simulink model "main_sim_claw_main_sf"  (Simulink 7.2)
settings: Solver=ode2  SolverMode=SingleTasking  StartTime=0.0  StopTime=tsim_max  FixedStep=dtsim  RelTol=1e-3
StopFcn:
  | %mkplt
undefined symbols (not defined in the file): assertion_time, dtsim, MACH, MACH_gain_mat, MACH_mass_IC, MACH_pos_IC, MACH_pqr_Bmat_IC, MACH_pqr_u_IC, MACH_quat_IC, MACH_throttle_IC, MACH_U_nom_IC, MACH_vel_Bmat_IC, MACH_vel_cvdnom_IC, MACH_vel_IC, MACH_vel_uold_IC, max_LOS_rate, target_pos_IC, target_vel_IC, trac_params, u_llim, u_ulim, use_variable_mass, x_trac_IC
libraries: model_lib x8, mach_lib x5, simulink x3, models x1, utility_lib x1
(part 1 of 2)
CloseFcn:
  | rtwprivate ssgencode ModelCloseRequest main
settings Model: Creator=E183308  LastModifiedBy=E183308  ModifiedComment=E700252 -- Tue Nov 11 13:33:23 2003 -- Version 1.2477  TunableVars=MACH_U_nom_IC,MACH_gain_mat,MACH_mass_IC,MACH_pos_IC,MACH_pqr_Bmat_IC,MACH_pqr_u_IC,MACH_quat_IC,MACH_throttle_IC,MACH_vel_Bmat_IC,MACH_vel_IC,MACH_vel_cvdnom_IC,MACH_vel_uold_IC  TunableVarsStorageClass=Auto,Auto,Auto,Auto,Auto,Auto,Auto,Auto,Auto,Auto,Auto,Auto  TunableVarsTypeQualifier=,,,,,,,,,,,  BufferReuse=off
settings DataIOCC: LimitDataPoints=off  SaveOutput=off  SaveTime=off  SignalLoggingName=sigsOut
settings OptimizationCC: BlockReduction=off  BooleanDataType=off  BufferReuse=off  EnforceIntegerDowncast=off  FoldNonRolledExpr=off  InitFltsAndDblsToZero=on
settings DebuggingCC: SaveWithParameterizedLinksMsg=none  SignalResolutionControl=TryResolveAllWithWarning  SolverPrmCheckMsg=none  InheritedTsInSrcMsg=none  MultiTaskDSMMsg=warning  MultiTaskCondExecSysMsg=none  StrictBusMsg=ErrorLevel1
settings HardwareCC: TargetEndianess=LittleEndian  TargetHWDeviceType=MATLAB Host  ProdEqTarget=off
settings SFSimCC: SFSimEcho=off
settings RTWCC: SystemTargetFile=rtwsfcn.tlc  TemplateMakefile=rtwsfcn_default_tmf  Description=S-function Target  ProcessScript=rtwsfcn_make_rtw_hook  IncludeERTFirstTime=on
settings STFCustomTargetCC: TargetFcnLib=ansi_tfl_tmw.mat  ModelReferenceCompliant=off  SystemTargetFile=rtwsfcn.tlc
settings CustomProperty: Value=on

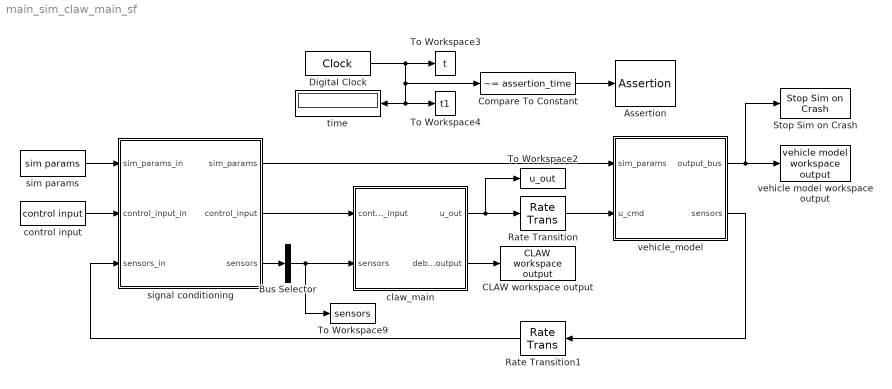
== system main_sim_claw_main_sf ==
  Assertion : Assertion  Enabled=on  AssertionFailFcn=assertioncb  StopWhenAssertionFail=off
  Bus Selector : BusSelector  OutputSignals=pqr,NED_dot,latlonh,e,accels_cg,nav_ok,u_meas,NED_wind,seeker  OutputAsBus=on
  CLAW workspace output : mach_lib/CLAW workspace output  SystemSampleTime=-1
  Compare To Constant : simulink/Logic and Bit Operations/Compare To Constant  SystemSampleTime=-1  relop=~=  const=assertion_time  LogicOutDataTypeMode=boolean  ZeroCross=off
  Digital Clock : DigitalClock  SampleTime=dtsim
  Rate Transition : RateTransition  X0=MACH_U_nom_IC
  Rate Transition1 : RateTransition  Orientation=left  OutPortSampleTime=MACH.dt
  Stop Sim on Crash : mach_lib/Stop Sim on Crash  SystemSampleTime=-1
  To Workspace2 : ToWorkspace  VariableName=u_out  SampleTime=MACH.dt  SaveFormat=Array
  To Workspace3 : ToWorkspace  VariableName=t  SampleTime=dtsim  SaveFormat=Array
  To Workspace4 : ToWorkspace  VariableName=t1  SampleTime=MACH.dt  SaveFormat=Array
  To Workspace9 : ToWorkspace  VariableName=sensors  SampleTime=MACH.dt  SaveFormat=Array
      settings: MaxDataPoints=1
  claw_main : Subsystem  mask{prm_to_disp=[1..10], sfcnParam1=MACH_U_nom_IC, sfcnParam2=MACH_gain_mat, sfcnParam3=MACH_mass_IC, sfcnParam4=MACH_pos_IC, sfcnParam5=MACH_pqr_Bmat_IC, sfcnParam6=MACH_pqr_u_IC, sfcnParam7=MACH_quat_IC, sfcnParam8=MACH_throttle_IC, sfcnParam9=MACH_vel_Bmat_IC, sfcnParam10=MACH_vel_IC, sfcnParam11=MACH_vel_cvdnom_IC, sfcnParam12=MACH_vel_uold_IC}
      mask prompts: prm_to_disp "Display S-function Parameters:"; sfcnParam1 "MACH_U_nom_IC:"; sfcnParam2 "MACH_gain_mat:"; sfcnParam3 "MACH_mass_IC:"; sfcnParam4 "MACH_pos_IC:"; sfcnParam5 "MACH_pqr_Bmat_IC:"; sfcnParam6 "MACH_pqr_u_IC:"; sfcnParam7 "MACH_quat_IC:"; sfcnParam8 "MACH_throttle_IC:"; sfcnParam9 "MACH_vel_Bmat_IC:"; sfcnParam10 "MACH_vel_IC:"; sfcnParam11 "MACH_vel_cvdnom_IC:"; sfcnParam12 "MACH_vel_uold_IC:"
      mask help: Real-Time Workshop generated S-function.
      mask Help: eval('feval(''rtwprivate'',''rtwhelpview'',''rtw_sfcn_block'')');
      mask StyleString: popup([1..10]|[11..12]),edit,edit,edit,edit,edit,edit,edit,edit,edit,edit,edit,edit
      mask CallbackString: slmaskprmdispcntrl(gcbh)||||||||||||
  control input : mach_lib/control input  SystemSampleTime=MACH.dt
  signal conditioning : Subsystem
  sim params : mach_lib/sim params  SystemSampleTime=-1
  time : Display
  vehicle model workspace output : mach_lib/vehicle model workspace output  SystemSampleTime=-1
  vehicle_model : Subsystem  TreatAsAtomicUnit=on
  wires:
  Digital Clock/1 -> To Workspace3/1, time/1, To Workspace4/1, Compare To Constant/1
  claw_main/1(u_out) -> Rate Transition/1, To Workspace2/1
  vehicle_model/2(sensors) -> Rate Transition1/1
  claw_main/2(debug_output) -> CLAW workspace output/1
  Rate Transition/1 -> vehicle_model/2(u_cmd)
  Bus Selector/1 -> To Workspace9/1, claw_main/2(sensors)
  vehicle_model/1(output_bus) -> vehicle model workspace output/1, Stop Sim on Crash/1
  Rate Transition1/1 -> signal conditioning/3(sensors_in)
  signal conditioning/3(sensors) -> Bus Selector/1
  signal conditioning/2(control_input) -> claw_main/1(control_input)
  control input/1 -> signal conditioning/2(control_input_in)
  sim params/1 -> signal conditioning/1(sim_params_in)
  signal conditioning/1(sim_params) -> vehicle_model/1(sim_params)
  Compare To Constant/1 -> Assertion/1

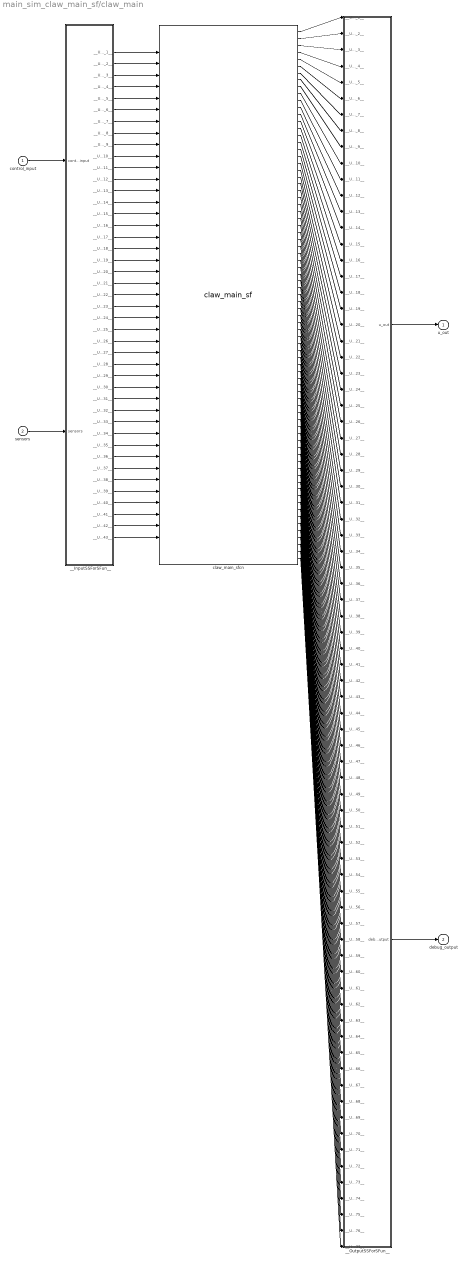
== system main_sim_claw_main_sf/claw_main ==
  control_input : Inport  OutDataType=sfix(16)  OutScaling=2^0
      settings: BusObject=control_input_bus
  sensors : Inport  Port=2  OutDataType=sfix(16)  OutScaling=2^0
  __InputSSForSFun__ : Subsystem
  __OutputSSForSFun__ : Subsystem
  claw_main_sfcn : S-Function  FunctionName=claw_main_sf  Parameters=sfcnParam1, sfcnParam2, sfcnParam3, sfcnParam4, sfcnParam5, sfcnParam6, sfcnParam7, sfcnParam8, sfcnParam9, sfcnParam10, sfcnParam11, sfcnParam12  SFunctionModules=""  EnableBusSupport=off  mask{rtw_sf_name=claw_main_sf, showVar=off, prm_to_disp=[1..10], sfcnParam1=sfcnParam1, sfcnParam2=sfcnParam2, sfcnParam3=sfcnParam3, sfcnParam4=sfcnParam4, sfcnParam5=sfcnParam5, sfcnParam6=sfcnParam6, sfcnParam7=sfcnParam7, sfcnParam8=sfcnParam8, sfcnParam9=sfcnParam9, sfcnParam10=sfcnParam10, sfcnParam11=sfcnParam11, sfcnParam12=sfcnParam12}
      mask prompts: rtw_sf_name "Generated S-function name (model_sf):"; showVar "Show module list"; prm_to_disp "Display S-function Parameters:"; sfcnParam1 "MACH_U_nom_IC:"; sfcnParam2 "MACH_gain_mat:"; sfcnParam3 "MACH_mass_IC:"; sfcnParam4 "MACH_pos_IC:"; sfcnParam5 "MACH_pqr_Bmat_IC:"; sfcnParam6 "MACH_pqr_u_IC:"; sfcnParam7 "MACH_quat_IC:"; sfcnParam8 "MACH_throttle_IC:"; sfcnParam9 "MACH_vel_Bmat_IC:"; sfcnParam10 "MACH_vel_IC:"; sfcnParam11 "MACH_vel_cvdnom_IC:"; sfcnParam12 "MACH_vel_uold_IC:"
      mask help: Real-Time Workshop generated S-function.
      mask init:
      | displist = '';
      | if ~strcmp(get_param(gcb, 'FunctionName'), rtw_sf_name);
      |   set_param(gcb, 'FunctionName', rtw_sf_name);
      | end
      | % Check if we are generating RTW code
      | rtw_mode = false;
      | if strcmpi(get_param(bdroot(gcb),'SimulationStatus'),'Initializing')
      | 	rtw_mode = strcmpi(get_param(bdroot(gcb),'BuildingRTWCode'),'on') && ...
      | 		~strcmpi(get_param(bdroot(gcb),'TargetStyle'),'SimulationTarget');
      | end
      | if showVar || rtw_mode
      | 	if exist('rtwsfunc') == 2 | exist('rtwsfunc') == 6
      | 		tmplist = rtwsfunc(rtw_sf_name,gcb);
      | 		tmplist = ['\nList of Modules:\n', tmplist];
      | 	elseif showVar
      | 		tmplist = '\nList of Modules:\nRTW not licensed\n';
      |  	end
      | end
      | if showVar
      |   displist = tmplist;
      | end
      settings: CopyFcn=|
      | if ~strcmp(get_param(gcb,'Linkstatus'),'none') && ...
      | ~strcmp(get_param(gcb,'Linkstatus'),'implicit')
      |   set_param(gcb,'LinkStatus','none');
      | end
      mask Help: eval('feval(''rtwprivate'',''rtwhelpview'',''rtw_sfcn_block'')');
      mask StyleString: edit,checkbox,popup([1..10]|[11..12]),edit,edit,edit,edit,edit,edit,edit,edit,edit,edit,edit,edit
      mask CallbackString: ||slmaskprmdispcntrl(gcbh)||||||||||||
      mask Display:
      | port_label('input',1,'command');
      | port_label('input',2,'full_surf_cmd');
      | port_label('input',3,'full_surf_ulim');
      | port_label('input',4,'full_surf_llim');
      | port_label('input',5,'full_surf_urlim');
      | port_label('input',6,'full_surf_lrlim');
      | port_label('input',7,'full_surf_lock');
      | port_label('input',8,'full_surf_pref_select');
      | port_label('input',9,'full_surf_pref');
      | port_label('input',10,'full_surf_pref_wght');
      | port_label('input',11,'CLAW_mode');
      | port_label('input',12,'engaged_sw');
      | port_label('input',13,'accel_submode');
      | port_label('input',14,'pre_takeoff_sw');
      | port_label('input',15,'reset_pos_sw');
      | port_label('input',16,'wind_est_sw');
      | port_label('input',17,'llh_input_sw');
      | port_label('input',18,'int_reset_sw');
      | port_label('input',19,'att_type');
      | port_label('input',20,'cam_rate_cmd_sw');
      | port_label('input',21,'full_surf_cmd_sw');
      | port_label('input',22,'enable_homing_sw');
      | port_label('input',23,'att_rate_cmd_sw');
      | port_label('input',24,'nav_enable_sw');
      | port_label('input',25,'enable_bb_sw');
      | port_label('input',26,'gain_set_sw');
      | port_label('input',27,'use_held_aero_obac_sw');
      | port_label('input',28,'Isp_sl');
      | port_label('input',29,'Isp_vacuum');
      | port_label('input',30,'throt_to_ff');
      | port_label('input',31,'pqr');
      | port_label('input',32,'NED_dot');
      | port_label('input',33,'latlonh');
      | port_label('input',34,'e');
      | port_label('input',35,'accels_cg');
      | port_label('input',36,'nav_ok');
      | port_label('input',37,'u_meas');
      | port_label('input',38,'NED_wind');
      | port_label('input',39,'LOS_rate');
      | port_label('input',40,'azimuth');
      | port_label('input',41,'elevation');
      | port_label('input',42,'Rground');
      | port_label('input',43,'Rslant');
      | port_label('output',1,'u_out');
      | port_label('output',2,'commandb');
      | port_label('output',3,'full_surf_cmdb');
      | port_label('output',4,'full_surf_ulimb');
      | port_label('output',5,'full_surf_llimb');
      | port_label('output',6,'full_surf_urlimb');
      | port_label('output',7,'full_surf_lrlimb');
      | port_label('output',8,'full_surf_lockb');
      | port_label('output',9,'full_surf_pref_selectb');
      | port_label('output',10,'full_surf_prefb');
      | port_label('output',11,'full_surf_pref_wghtb');
      | port_label('output',12,'CLAW_modeb');
      | port_label('output',13,'engaged_swb');
      | port_label('output',14,'accel_submodeb');
      | port_label('output',15,'pre_takeoff_swb');
      | port_label('output',16,'reset_pos_swb');
      | port_label('output',17,'wind_est_swb');
      | port_label('output',18,'llh_input_swb');
      | port_label('output',19,'int_reset_swb');
      | port_label('output',20,'att_typeb');
      | port_label('output',21,'cam_rate_cmd_swb');
      | port_label('output',22,'full_surf_cmd_swb');
      | port_label('output',23,'enable_homing_swb');
      | port_label('output',24,'att_rate_cmd_swb');
      | port_label('output',25,'nav_enable_swb');
      | port_label('output',26,'enable_bb_swb');
      | port_label('output',27,'gain_set_swb');
      | port_label('output',28,'use_held_aero_obac_swb');
      | port_label('output',29,'Isp_slb');
      | port_label('output',30,'Isp_vacuumb');
      | port_label('output',31,'throt_to_ffb');
      | port_label('output',32,'cvdex_smn');
      | port_label('output',33,'lambda');
      | port_label('output',34,'solve_dat');
      | port_label('output',35,'cvdex');
      | port_label('output',36,'cvc');
      | port_label('output',37,'integ');
      | port_label('output',38,'cv');
      | port_label('output',39,'cvdnom');
      | port_label('output',40,'Bmat');
      | port_label('output',41,'u_ulim');
      | port_label('output',42,'u_llim');
      | port_label('output',43,'u_pref');
      | port_label('output',44,'bb_debug');
      | port_label('output',45,'cvdexb');
      | port_label('output',46,'integb');
      | port_label('output',47,'cvcb');
      | port_label('output',48,'cvb');
      | port_label('output',49,'tiltcam_cmds');
      | port_label('output',50,'rpy_cmds');
      | port_label('output',51,'mab_cmds');
      | port_label('output',52,'cvdexa');
      | port_label('output',53,'lambdab');
      | port_label('output',54,'solve_datb');
      | port_label('output',55,'intega');
      | port_label('output',56,'cvca');
      | port_label('output',57,'cva');
      | port_label('output',58,'cvdnomb');
      | port_label('output',59,'Bmatb');
      | port_label('output',60,'Bmat_fltpath');
      | port_label('output',61,'u_ulimb');
      | port_label('output',62,'u_llimb');
      | port_label('output',63,'cvdex_fltpath');
      | port_label('output',64,'cvdexc');
      | port_label('output',65,'integc');
      | port_label('output',66,'cvcc');
      | port_label('output',67,'cvd');
      | port_label('output',68,'cvdex_fltpathb');
      | port_label('output',69,'w_est');
      | port_label('output',70,'NED_wind_ex');
      | port_label('output',71,'uvw_wind');
      | port_label('output',72,'uvw_rw_est');
      | port_label('output',73,'accels');
      | port_label('output',74,'att_typea');
      | port_label('output',75,'mass');
      | port_label('output',76,'enable_bb');
      | port_label('output',77,'gain_set');
  u_out : Outport  OutDataType=sfix(16)  OutScaling=2^0
  debug_output : Outport  Port=2  OutDataType=sfix(16)  OutScaling=2^0
  wires:
  control_input/1 -> __InputSSForSFun__/1(control_input)
  sensors/1 -> __InputSSForSFun__/2(sensors)
  __InputSSForSFun__/1(__UniqueOutportName__1__) -> claw_main_sfcn/1
  __InputSSForSFun__/2(__UniqueOutportName__2__) -> claw_main_sfcn/2
  __InputSSForSFun__/3(__UniqueOutportName__3__) -> claw_main_sfcn/3
  __InputSSForSFun__/4(__UniqueOutportName__4__) -> claw_main_sfcn/4
  __InputSSForSFun__/5(__UniqueOutportName__5__) -> claw_main_sfcn/5
  __InputSSForSFun__/6(__UniqueOutportName__6__) -> claw_main_sfcn/6
  __InputSSForSFun__/7(__UniqueOutportName__7__) -> claw_main_sfcn/7
  __InputSSForSFun__/8(__UniqueOutportName__8__) -> claw_main_sfcn/8
  __InputSSForSFun__/9(__UniqueOutportName__9__) -> claw_main_sfcn/9
  __InputSSForSFun__/10(__UniqueOutportName__10__) -> claw_main_sfcn/10
  __InputSSForSFun__/11(__UniqueOutportName__11__) -> claw_main_sfcn/11
  __InputSSForSFun__/12(__UniqueOutportName__12__) -> claw_main_sfcn/12
  __InputSSForSFun__/13(__UniqueOutportName__13__) -> claw_main_sfcn/13
  __InputSSForSFun__/14(__UniqueOutportName__14__) -> claw_main_sfcn/14
  __InputSSForSFun__/15(__UniqueOutportName__15__) -> claw_main_sfcn/15
  __InputSSForSFun__/16(__UniqueOutportName__16__) -> claw_main_sfcn/16
  __InputSSForSFun__/17(__UniqueOutportName__17__) -> claw_main_sfcn/17
  __InputSSForSFun__/18(__UniqueOutportName__18__) -> claw_main_sfcn/18
  __InputSSForSFun__/19(__UniqueOutportName__19__) -> claw_main_sfcn/19
  __InputSSForSFun__/20(__UniqueOutportName__20__) -> claw_main_sfcn/20
  __InputSSForSFun__/21(__UniqueOutportName__21__) -> claw_main_sfcn/21
  __InputSSForSFun__/22(__UniqueOutportName__22__) -> claw_main_sfcn/22
  __InputSSForSFun__/23(__UniqueOutportName__23__) -> claw_main_sfcn/23
  __InputSSForSFun__/24(__UniqueOutportName__24__) -> claw_main_sfcn/24
  __InputSSForSFun__/25(__UniqueOutportName__25__) -> claw_main_sfcn/25
  __InputSSForSFun__/26(__UniqueOutportName__26__) -> claw_main_sfcn/26
  __InputSSForSFun__/27(__UniqueOutportName__27__) -> claw_main_sfcn/27
  __InputSSForSFun__/28(__UniqueOutportName__28__) -> claw_main_sfcn/28
  __InputSSForSFun__/29(__UniqueOutportName__29__) -> claw_main_sfcn/29
  __InputSSForSFun__/30(__UniqueOutportName__30__) -> claw_main_sfcn/30
  __InputSSForSFun__/31(__UniqueOutportName__31__) -> claw_main_sfcn/31
  __InputSSForSFun__/32(__UniqueOutportName__32__) -> claw_main_sfcn/32
  __InputSSForSFun__/33(__UniqueOutportName__33__) -> claw_main_sfcn/33
  __InputSSForSFun__/34(__UniqueOutportName__34__) -> claw_main_sfcn/34
  __InputSSForSFun__/35(__UniqueOutportName__35__) -> claw_main_sfcn/35
  __InputSSForSFun__/36(__UniqueOutportName__36__) -> claw_main_sfcn/36
  __InputSSForSFun__/37(__UniqueOutportName__37__) -> claw_main_sfcn/37
  __InputSSForSFun__/38(__UniqueOutportName__38__) -> claw_main_sfcn/38
  __InputSSForSFun__/39(__UniqueOutportName__39__) -> claw_main_sfcn/39
  __InputSSForSFun__/40(__UniqueOutportName__40__) -> claw_main_sfcn/40
  __InputSSForSFun__/41(__UniqueOutportName__41__) -> claw_main_sfcn/41
  __InputSSForSFun__/42(__UniqueOutportName__42__) -> claw_main_sfcn/42
  __InputSSForSFun__/43(__UniqueOutportName__43__) -> claw_main_sfcn/43
  claw_main_sfcn/1 -> __OutputSSForSFun__/1(__UniqueInportName__1__)
  claw_main_sfcn/2 -> __OutputSSForSFun__/2(__UniqueInportName__2__)
  claw_main_sfcn/3 -> __OutputSSForSFun__/3(__UniqueInportName__3__)
  claw_main_sfcn/4 -> __OutputSSForSFun__/4(__UniqueInportName__4__)
  claw_main_sfcn/5 -> __OutputSSForSFun__/5(__UniqueInportName__5__)
  claw_main_sfcn/6 -> __OutputSSForSFun__/6(__UniqueInportName__6__)
  claw_main_sfcn/7 -> __OutputSSForSFun__/7(__UniqueInportName__7__)
  claw_main_sfcn/8 -> __OutputSSForSFun__/8(__UniqueInportName__8__)
  claw_main_sfcn/9 -> __OutputSSForSFun__/9(__UniqueInportName__9__)
  claw_main_sfcn/10 -> __OutputSSForSFun__/10(__UniqueInportName__10__)
  claw_main_sfcn/11 -> __OutputSSForSFun__/11(__UniqueInportName__11__)
  claw_main_sfcn/12 -> __OutputSSForSFun__/12(__UniqueInportName__12__)
  claw_main_sfcn/13 -> __OutputSSForSFun__/13(__UniqueInportName__13__)
  claw_main_sfcn/14 -> __OutputSSForSFun__/14(__UniqueInportName__14__)
  claw_main_sfcn/15 -> __OutputSSForSFun__/15(__UniqueInportName__15__)
  claw_main_sfcn/16 -> __OutputSSForSFun__/16(__UniqueInportName__16__)
  claw_main_sfcn/17 -> __OutputSSForSFun__/17(__UniqueInportName__17__)
  claw_main_sfcn/18 -> __OutputSSForSFun__/18(__UniqueInportName__18__)
  claw_main_sfcn/19 -> __OutputSSForSFun__/19(__UniqueInportName__19__)
  claw_main_sfcn/20 -> __OutputSSForSFun__/20(__UniqueInportName__20__)
  claw_main_sfcn/21 -> __OutputSSForSFun__/21(__UniqueInportName__21__)
  claw_main_sfcn/22 -> __OutputSSForSFun__/22(__UniqueInportName__22__)
  claw_main_sfcn/23 -> __OutputSSForSFun__/23(__UniqueInportName__23__)
  claw_main_sfcn/24 -> __OutputSSForSFun__/24(__UniqueInportName__24__)
  claw_main_sfcn/25 -> __OutputSSForSFun__/25(__UniqueInportName__25__)
  claw_main_sfcn/26 -> __OutputSSForSFun__/26(__UniqueInportName__26__)
  claw_main_sfcn/27 -> __OutputSSForSFun__/27(__UniqueInportName__27__)
  claw_main_sfcn/28 -> __OutputSSForSFun__/28(__UniqueInportName__28__)
  claw_main_sfcn/29 -> __OutputSSForSFun__/29(__UniqueInportName__29__)
  claw_main_sfcn/30 -> __OutputSSForSFun__/30(__UniqueInportName__30__)
  claw_main_sfcn/31 -> __OutputSSForSFun__/31(__UniqueInportName__31__)
  claw_main_sfcn/32 -> __OutputSSForSFun__/32(__UniqueInportName__32__)
  claw_main_sfcn/33 -> __OutputSSForSFun__/33(__UniqueInportName__33__)
  claw_main_sfcn/34 -> __OutputSSForSFun__/34(__UniqueInportName__34__)
  claw_main_sfcn/35 -> __OutputSSForSFun__/35(__UniqueInportName__35__)
  claw_main_sfcn/36 -> __OutputSSForSFun__/36(__UniqueInportName__36__)
  claw_main_sfcn/37 -> __OutputSSForSFun__/37(__UniqueInportName__37__)
  claw_main_sfcn/38 -> __OutputSSForSFun__/38(__UniqueInportName__38__)
  claw_main_sfcn/39 -> __OutputSSForSFun__/39(__UniqueInportName__39__)
  claw_main_sfcn/40 -> __OutputSSForSFun__/40(__UniqueInportName__40__)
  claw_main_sfcn/41 -> __OutputSSForSFun__/41(__UniqueInportName__41__)
  claw_main_sfcn/42 -> __OutputSSForSFun__/42(__UniqueInportName__42__)
  claw_main_sfcn/43 -> __OutputSSForSFun__/43(__UniqueInportName__43__)
  claw_main_sfcn/44 -> __OutputSSForSFun__/44(__UniqueInportName__44__)
  claw_main_sfcn/45 -> __OutputSSForSFun__/45(__UniqueInportName__45__)
  claw_main_sfcn/46 -> __OutputSSForSFun__/46(__UniqueInportName__46__)
  claw_main_sfcn/47 -> __OutputSSForSFun__/47(__UniqueInportName__47__)
  claw_main_sfcn/48 -> __OutputSSForSFun__/48(__UniqueInportName__48__)
  claw_main_sfcn/49 -> __OutputSSForSFun__/49(__UniqueInportName__49__)
  claw_main_sfcn/50 -> __OutputSSForSFun__/50(__UniqueInportName__50__)
  claw_main_sfcn/51 -> __OutputSSForSFun__/51(__UniqueInportName__51__)
  claw_main_sfcn/52 -> __OutputSSForSFun__/52(__UniqueInportName__52__)
  claw_main_sfcn/53 -> __OutputSSForSFun__/53(__UniqueInportName__53__)
  claw_main_sfcn/54 -> __OutputSSForSFun__/54(__UniqueInportName__54__)
  claw_main_sfcn/55 -> __OutputSSForSFun__/55(__UniqueInportName__55__)
  claw_main_sfcn/56 -> __OutputSSForSFun__/56(__UniqueInportName__56__)
  claw_main_sfcn/57 -> __OutputSSForSFun__/57(__UniqueInportName__57__)
  claw_main_sfcn/58 -> __OutputSSForSFun__/58(__UniqueInportName__58__)
  claw_main_sfcn/59 -> __OutputSSForSFun__/59(__UniqueInportName__59__)
  claw_main_sfcn/60 -> __OutputSSForSFun__/60(__UniqueInportName__60__)
  claw_main_sfcn/61 -> __OutputSSForSFun__/61(__UniqueInportName__61__)
  claw_main_sfcn/62 -> __OutputSSForSFun__/62(__UniqueInportName__62__)
  claw_main_sfcn/63 -> __OutputSSForSFun__/63(__UniqueInportName__63__)
  claw_main_sfcn/64 -> __OutputSSForSFun__/64(__UniqueInportName__64__)
  claw_main_sfcn/65 -> __OutputSSForSFun__/65(__UniqueInportName__65__)
  claw_main_sfcn/66 -> __OutputSSForSFun__/66(__UniqueInportName__66__)
  claw_main_sfcn/67 -> __OutputSSForSFun__/67(__UniqueInportName__67__)
  claw_main_sfcn/68 -> __OutputSSForSFun__/68(__UniqueInportName__68__)
  claw_main_sfcn/69 -> __OutputSSForSFun__/69(__UniqueInportName__69__)
  claw_main_sfcn/70 -> __OutputSSForSFun__/70(__UniqueInportName__70__)
  claw_main_sfcn/71 -> __OutputSSForSFun__/71(__UniqueInportName__71__)
  claw_main_sfcn/72 -> __OutputSSForSFun__/72(__UniqueInportName__72__)
  claw_main_sfcn/73 -> __OutputSSForSFun__/73(__UniqueInportName__73__)
  claw_main_sfcn/74 -> __OutputSSForSFun__/74(__UniqueInportName__74__)
  claw_main_sfcn/75 -> __OutputSSForSFun__/75(__UniqueInportName__75__)
  claw_main_sfcn/76 -> __OutputSSForSFun__/76(__UniqueInportName__76__)
  claw_main_sfcn/77 -> __OutputSSForSFun__/77(__UniqueInportName__77__)
  __OutputSSForSFun__/1(u_out) -> u_out/1
  __OutputSSForSFun__/2(debug_output) -> debug_output/1

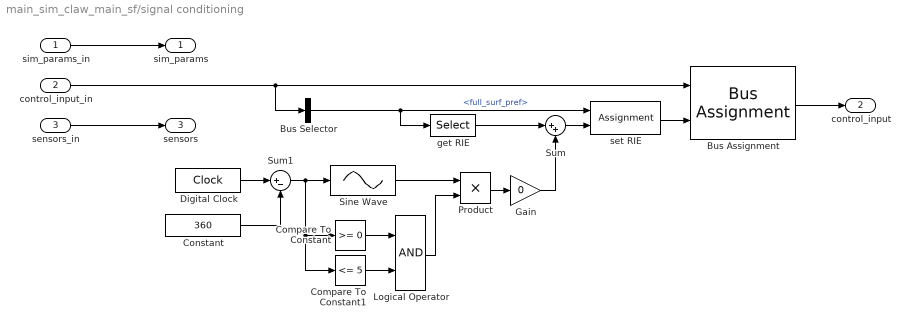
== system main_sim_claw_main_sf/signal conditioning ==
  sim_params_in : Inport  OutDataType=sfix(16)  OutScaling=2^0
  control_input_in : Inport  Port=2  OutDataType=sfix(16)  OutScaling=2^0
  sensors_in : Inport  Port=3  OutDataType=sfix(16)  OutScaling=2^0
  Bus Assignment : BusAssignment  AssignedSignals=full_surf.full_surf_pref
  Bus Selector : BusSelector  OutputSignals=full_surf.full_surf_pref
  Compare To Constant : simulink/Logic and Bit Operations/Compare To Constant  SystemSampleTime=-1  relop=>=  const=0  LogicOutDataTypeMode=boolean  ZeroCross=off
  Compare To Constant1 : simulink/Logic and Bit Operations/Compare To Constant  SystemSampleTime=-1  relop=<=  const=5  LogicOutDataTypeMode=boolean  ZeroCross=off
  Constant : Constant  Value=360  OutDataType=sfix(16)  OutScaling=2^0
  Digital Clock : DigitalClock  SampleTime=MACH.dt
  Gain : Gain  Gain=0  ParameterDataType=sfix(16)  ParameterScaling=2^0  OutDataType=sfix(16)  OutScaling=2^0
  Logical Operator : Logic  AllPortsSameDT=off
  Product : Product  OutDataType=sfix(16)  OutScaling=2^0  RndMeth=Zero
  Sine Wave : Sin  TimeSource=Use external signal  Amplitude=5  Frequency=2*pi  SampleTime=0
  Sum : Sum  Inputs=|++  OutDataType=sfix(16)  OutScaling=2^0
  Sum1 : Sum  Inputs=|+-  OutDataType=sfix(16)  OutScaling=2^0
  get RIE : Selector  InputPortWidth=MACH.num_u  IndexOptions=Index vector (dialog)  Indices=MACH.vane_idx(1)  OutputSizes=1
  set RIE : Assignment  IndexOptions=Index vector (dialog)  Indices=MACH.vane_idx(1)  OutputSizes=[1 1]
  sim_params : Outport  OutDataType=sfix(16)  OutScaling=2^0
  control_input : Outport  Port=2  OutDataType=sfix(16)  OutScaling=2^0
  sensors : Outport  Port=3  OutDataType=sfix(16)  OutScaling=2^0
  wires:
  sim_params_in/1 -> sim_params/1
  control_input_in/1 -> Bus Assignment/1, Bus Selector/1
  sensors_in/1 -> sensors/1
  set RIE/1 -> Bus Assignment/2
  Sum/1 -> set RIE/2
  Bus Selector/1 -> set RIE/1, get RIE/1  "<full_surf_pref>"
  get RIE/1 -> Sum/1
  Digital Clock/1 -> Sum1/1
  Constant/1 -> Sum1/2
  Sum1/1 -> Sine Wave/1, Compare To Constant/1, Compare To Constant1/1
  Compare To Constant/1 -> Logical Operator/1
  Compare To Constant1/1 -> Logical Operator/2
  Logical Operator/1 -> Product/2
  Sine Wave/1 -> Product/1
  Product/1 -> Gain/1
  Bus Assignment/1 -> control_input/1
  Gain/1 -> Sum/2

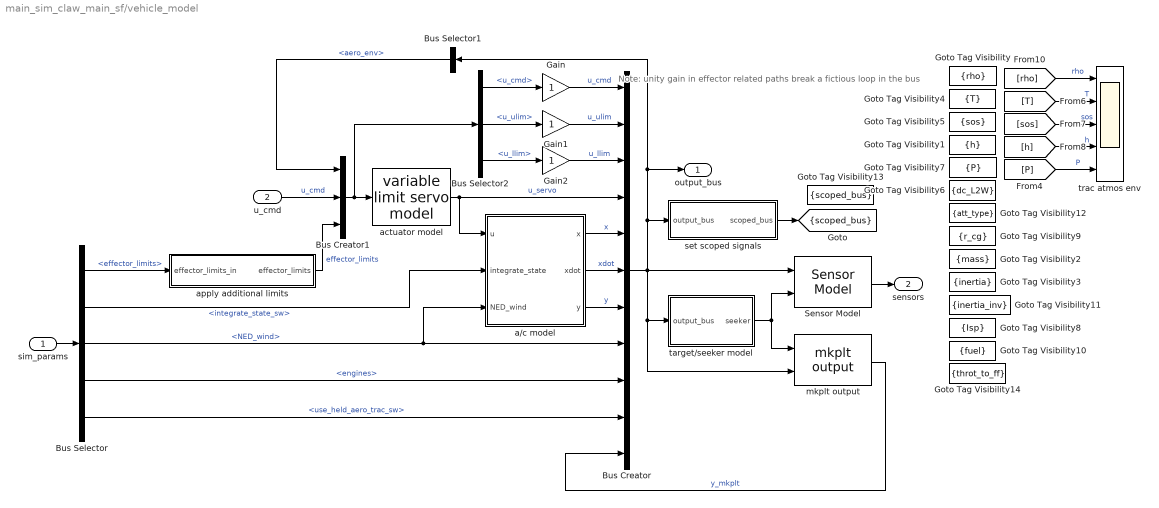
== system main_sim_claw_main_sf/vehicle_model ==
  note: Note: unity gain in effector related paths
      | break a fictious loop in the bus
  sim_params : Inport  OutDataType=sfix(16)  OutScaling=2^0
  u_cmd : Inport  Port=2  OutDataType=sfix(16)  OutScaling=2^0
  Bus Creator : BusCreator  Inputs=11
  Bus Creator1 : BusCreator  Inputs=3
  Bus Selector : BusSelector  OutputSignals=effector_limits,integrate_state_sw,NED_wind,engines,use_held_aero_trac_sw
  Bus Selector1 : BusSelector  Orientation=left  OutputSignals=y.aero_env
  Bus Selector2 : BusSelector  OutputSignals=u_cmd,effector_limits.u_ulim,effector_limits.u_llim
  Gain : Gain  ParameterDataType=sfix(16)  ParameterScaling=2^0  OutDataType=sfix(16)  OutScaling=2^0
  Gain1 : Gain  ParameterDataType=sfix(16)  ParameterScaling=2^0  OutDataType=sfix(16)  OutScaling=2^0
  Gain2 : Gain  ParameterDataType=sfix(16)  ParameterScaling=2^0  OutDataType=sfix(16)  OutScaling=2^0
  Goto Tag Visibility : GotoTagVisibility  GotoTag=rho
  Goto Tag Visibility1 : GotoTagVisibility  GotoTag=h
  Goto Tag Visibility10 : GotoTagVisibility  GotoTag=fuel
  Goto Tag Visibility11 : GotoTagVisibility  GotoTag=inertia_inv
  Goto Tag Visibility12 : GotoTagVisibility  GotoTag=att_type
  Goto Tag Visibility13 : GotoTagVisibility  GotoTag=scoped_bus
  Goto Tag Visibility14 : GotoTagVisibility  GotoTag=throt_to_ff
  Goto Tag Visibility2 : GotoTagVisibility  GotoTag=mass
  Goto Tag Visibility3 : GotoTagVisibility  GotoTag=inertia
  Goto Tag Visibility4 : GotoTagVisibility  GotoTag=T
  Goto Tag Visibility5 : GotoTagVisibility  GotoTag=sos
  Goto Tag Visibility6 : GotoTagVisibility  GotoTag=dc_L2W
  Goto Tag Visibility7 : GotoTagVisibility  GotoTag=P
  Goto Tag Visibility8 : GotoTagVisibility  GotoTag=Isp
  Goto Tag Visibility9 : GotoTagVisibility  GotoTag=r_cg
  Sensor Model : model_lib/Sensor Model  SystemSampleTime=-1
  a/c model : Subsystem
  actuator model : model_lib/variable limit servo model  SystemSampleTime=-1
  apply additional limits : Subsystem
  mkplt output : model_lib/mkplt output  SystemSampleTime=-1
  set scoped signals : Subsystem
  target/seeker model : Subsystem
  trac atmos env : Scope  NumInputPorts=5
      settings: YMin=-5~-5~-5~-5~-5  YMax=5~5~5~5~5
  output_bus : Outport  OutDataType=sfix(16)  OutScaling=2^0
  sensors : Outport  Port=2  OutDataType=sfix(16)  OutScaling=2^0
  tag scope: scoped_bus=scoped
  wires:
  actuator model/1 -> a/c model/1(u), Bus Creator/4  "u_servo"
  Sensor Model/1 -> sensors/1
  Bus Selector/3 -> Bus Creator/8, a/c model/3(NED_wind)  "<NED_wind>"
  [h] -> trac atmos env/4  "h"
  [sos] -> trac atmos env/3  "sos"
  [T] -> trac atmos env/2  "T"
  [rho] -> trac atmos env/1  "rho"
  [P] -> trac atmos env/5  "P"
  target/seeker model/1(seeker) -> Sensor Model/2, mkplt output/1
  a/c model/1(x) -> Bus Creator/5  "x"
  a/c model/2(xdot) -> Bus Creator/6  "xdot"
  a/c model/3(y) -> Bus Creator/7  "y"
  Bus Creator/1 -> set scoped signals/1(output_bus), output_bus/1, Bus Selector1/1, target/seeker model/1(output_bus), mkplt output/2, Sensor Model/1
  sim_params/1 -> Bus Selector/1
  set scoped signals/1(scoped_bus) -> [scoped_bus]
  Bus Selector/4 -> Bus Creator/9  "<engines>"
  mkplt output/1 -> Bus Creator/11  "y_mkplt"
  Bus Selector/5 -> Bus Creator/10  "<use_held_aero_trac_sw>"
  Bus Creator1/1 -> actuator model/1, Bus Selector2/1
  Bus Selector1/1 -> Bus Creator1/1  "<aero_env>"
  u_cmd/1 -> Bus Creator1/2  "u_cmd"
  Bus Selector2/1 -> Gain/1  "<u_cmd>"
  Bus Selector2/2 -> Gain1/1  "<u_ulim>"
  Bus Selector2/3 -> Gain2/1  "<u_llim>"
  Gain/1 -> Bus Creator/1  "u_cmd"
  Gain1/1 -> Bus Creator/2  "u_ulim"
  Gain2/1 -> Bus Creator/3  "u_llim"
  Bus Selector/2 -> a/c model/2(integrate_state)  "<integrate_state_sw>"
  Bus Selector/1 -> apply additional limits/1(effector_limits_in)  "<effector_limits>"
  apply additional limits/1(effector_limits) -> Bus Creator1/3  "effector_limits"

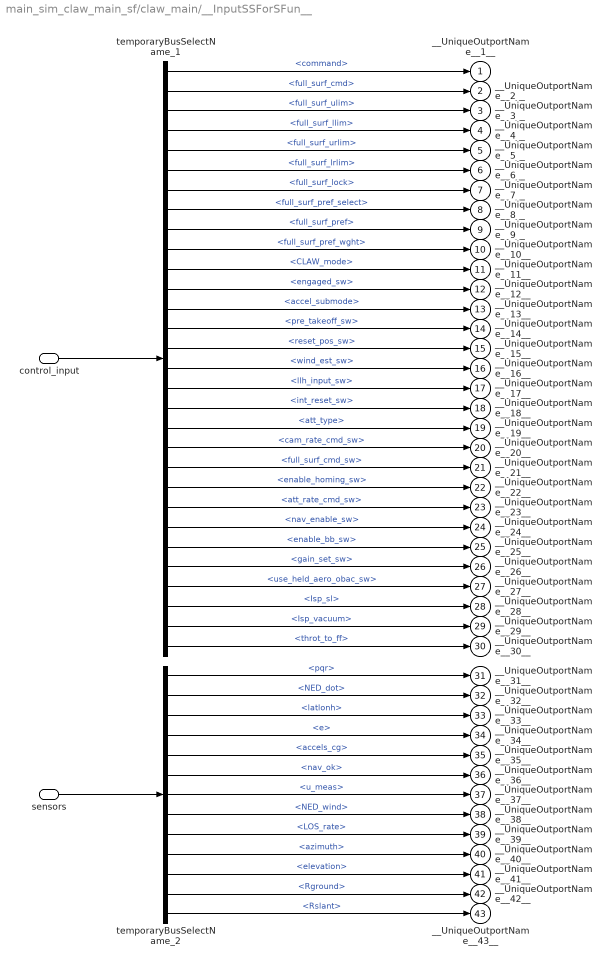
== system main_sim_claw_main_sf/claw_main/__InputSSForSFun__ ==
  control_input : Inport  OutDataType=sfix(16)  OutScaling=2^0
      settings: BusObject=control_input_bus
  sensors : Inport  Port=2  OutDataType=sfix(16)  OutScaling=2^0
  temporaryBusSelectName_1 : BusSelector  OutputSignals=command,full_surf.full_surf_cmd,full_surf.full_surf_ulim,full_surf.full_surf_llim,full_surf.full_surf_urlim,full_surf.full_surf_lrlim,full_surf.full_surf_lock,full_surf.full_surf_pref_select,full_surf.full_surf_pref,full_surf.full_surf_pref_wght,mode_sw.CLAW_mode,mode_sw.engaged_sw,mode_sw.accel_submode,mode_sw.pre_takeoff_sw,mode_sw.reset_pos_sw,mode_sw.wind_est_sw,mode_sw.llh_input_sw,mode_sw.int_reset_sw,mode_sw.att_type,mode_sw.cam_rate_cmd_sw,mode_sw.full_surf_cmd_sw,mode_sw.enable_homing_sw,mode_sw.att_rate_cmd_sw,mode_sw.nav_enable_sw,mode_sw.enable_bb_sw,mode_sw.gain_set_sw,mode_sw.use_held_aero_obac_sw,engines.Isp_sl,engines.Isp_vacuum,engines.throt_to_ff
  temporaryBusSelectName_2 : BusSelector  OutputSignals=pqr,NED_dot,latlonh,e,accels_cg,nav_ok,u_meas,NED_wind,seeker.LOS_rate,seeker.aux_info.azimuth,seeker.aux_info.elevation,seeker.aux_info.Rground,seeker.aux_info.Rslant
  __UniqueOutportName__1__ : Outport
  __UniqueOutportName__2__ : Outport  Port=2
  __UniqueOutportName__3__ : Outport  Port=3
  __UniqueOutportName__4__ : Outport  Port=4
  __UniqueOutportName__5__ : Outport  Port=5
  __UniqueOutportName__6__ : Outport  Port=6
  __UniqueOutportName__7__ : Outport  Port=7
  __UniqueOutportName__8__ : Outport  Port=8
  __UniqueOutportName__9__ : Outport  Port=9
  __UniqueOutportName__10__ : Outport  Port=10
  __UniqueOutportName__11__ : Outport  Port=11
  __UniqueOutportName__12__ : Outport  Port=12
  __UniqueOutportName__13__ : Outport  Port=13
  __UniqueOutportName__14__ : Outport  Port=14
  __UniqueOutportName__15__ : Outport  Port=15
  __UniqueOutportName__16__ : Outport  Port=16
  __UniqueOutportName__17__ : Outport  Port=17
  __UniqueOutportName__18__ : Outport  Port=18
  __UniqueOutportName__19__ : Outport  Port=19
  __UniqueOutportName__20__ : Outport  Port=20
  __UniqueOutportName__21__ : Outport  Port=21
  __UniqueOutportName__22__ : Outport  Port=22
  __UniqueOutportName__23__ : Outport  Port=23
  __UniqueOutportName__24__ : Outport  Port=24
  __UniqueOutportName__25__ : Outport  Port=25
  __UniqueOutportName__26__ : Outport  Port=26
  __UniqueOutportName__27__ : Outport  Port=27
  __UniqueOutportName__28__ : Outport  Port=28
  __UniqueOutportName__29__ : Outport  Port=29
  __UniqueOutportName__30__ : Outport  Port=30
  __UniqueOutportName__31__ : Outport  Port=31
  __UniqueOutportName__32__ : Outport  Port=32
  __UniqueOutportName__33__ : Outport  Port=33
  __UniqueOutportName__34__ : Outport  Port=34
  __UniqueOutportName__35__ : Outport  Port=35
  __UniqueOutportName__36__ : Outport  Port=36
  __UniqueOutportName__37__ : Outport  Port=37
  __UniqueOutportName__38__ : Outport  Port=38
  __UniqueOutportName__39__ : Outport  Port=39
  __UniqueOutportName__40__ : Outport  Port=40
  __UniqueOutportName__41__ : Outport  Port=41
  __UniqueOutportName__42__ : Outport  Port=42
  __UniqueOutportName__43__ : Outport  Port=43
  wires:
  control_input/1 -> temporaryBusSelectName_1/1
  sensors/1 -> temporaryBusSelectName_2/1
  temporaryBusSelectName_1/1 -> __UniqueOutportName__1__/1  "<command>"
  temporaryBusSelectName_1/2 -> __UniqueOutportName__2__/1  "<full_surf_cmd>"
  temporaryBusSelectName_1/3 -> __UniqueOutportName__3__/1  "<full_surf_ulim>"
  temporaryBusSelectName_1/4 -> __UniqueOutportName__4__/1  "<full_surf_llim>"
  temporaryBusSelectName_1/5 -> __UniqueOutportName__5__/1  "<full_surf_urlim>"
  temporaryBusSelectName_1/6 -> __UniqueOutportName__6__/1  "<full_surf_lrlim>"
  temporaryBusSelectName_1/7 -> __UniqueOutportName__7__/1  "<full_surf_lock>"
  temporaryBusSelectName_1/8 -> __UniqueOutportName__8__/1  "<full_surf_pref_select>"
  temporaryBusSelectName_1/9 -> __UniqueOutportName__9__/1  "<full_surf_pref>"
  temporaryBusSelectName_1/10 -> __UniqueOutportName__10__/1  "<full_surf_pref_wght>"
  temporaryBusSelectName_1/11 -> __UniqueOutportName__11__/1  "<CLAW_mode>"
  temporaryBusSelectName_1/12 -> __UniqueOutportName__12__/1  "<engaged_sw>"
  temporaryBusSelectName_1/13 -> __UniqueOutportName__13__/1  "<accel_submode>"
  temporaryBusSelectName_1/14 -> __UniqueOutportName__14__/1  "<pre_takeoff_sw>"
  temporaryBusSelectName_1/15 -> __UniqueOutportName__15__/1  "<reset_pos_sw>"
  temporaryBusSelectName_1/16 -> __UniqueOutportName__16__/1  "<wind_est_sw>"
  temporaryBusSelectName_1/17 -> __UniqueOutportName__17__/1  "<llh_input_sw>"
  temporaryBusSelectName_1/18 -> __UniqueOutportName__18__/1  "<int_reset_sw>"
  temporaryBusSelectName_1/19 -> __UniqueOutportName__19__/1  "<att_type>"
  temporaryBusSelectName_1/20 -> __UniqueOutportName__20__/1  "<cam_rate_cmd_sw>"
  temporaryBusSelectName_1/21 -> __UniqueOutportName__21__/1  "<full_surf_cmd_sw>"
  temporaryBusSelectName_1/22 -> __UniqueOutportName__22__/1  "<enable_homing_sw>"
  temporaryBusSelectName_1/23 -> __UniqueOutportName__23__/1  "<att_rate_cmd_sw>"
  temporaryBusSelectName_1/24 -> __UniqueOutportName__24__/1  "<nav_enable_sw>"
  temporaryBusSelectName_1/25 -> __UniqueOutportName__25__/1  "<enable_bb_sw>"
  temporaryBusSelectName_1/26 -> __UniqueOutportName__26__/1  "<gain_set_sw>"
  temporaryBusSelectName_1/27 -> __UniqueOutportName__27__/1  "<use_held_aero_obac_sw>"
  temporaryBusSelectName_1/28 -> __UniqueOutportName__28__/1  "<Isp_sl>"
  temporaryBusSelectName_1/29 -> __UniqueOutportName__29__/1  "<Isp_vacuum>"
  temporaryBusSelectName_1/30 -> __UniqueOutportName__30__/1  "<throt_to_ff>"
  temporaryBusSelectName_2/1 -> __UniqueOutportName__31__/1  "<pqr>"
  temporaryBusSelectName_2/2 -> __UniqueOutportName__32__/1  "<NED_dot>"
  temporaryBusSelectName_2/3 -> __UniqueOutportName__33__/1  "<latlonh>"
  temporaryBusSelectName_2/4 -> __UniqueOutportName__34__/1  "<e>"
  temporaryBusSelectName_2/5 -> __UniqueOutportName__35__/1  "<accels_cg>"
  temporaryBusSelectName_2/6 -> __UniqueOutportName__36__/1  "<nav_ok>"
  temporaryBusSelectName_2/7 -> __UniqueOutportName__37__/1  "<u_meas>"
  temporaryBusSelectName_2/8 -> __UniqueOutportName__38__/1  "<NED_wind>"
  temporaryBusSelectName_2/9 -> __UniqueOutportName__39__/1  "<LOS_rate>"
  temporaryBusSelectName_2/10 -> __UniqueOutportName__40__/1  "<azimuth>"
  temporaryBusSelectName_2/11 -> __UniqueOutportName__41__/1  "<elevation>"
  temporaryBusSelectName_2/12 -> __UniqueOutportName__42__/1  "<Rground>"
  temporaryBusSelectName_2/13 -> __UniqueOutportName__43__/1  "<Rslant>"

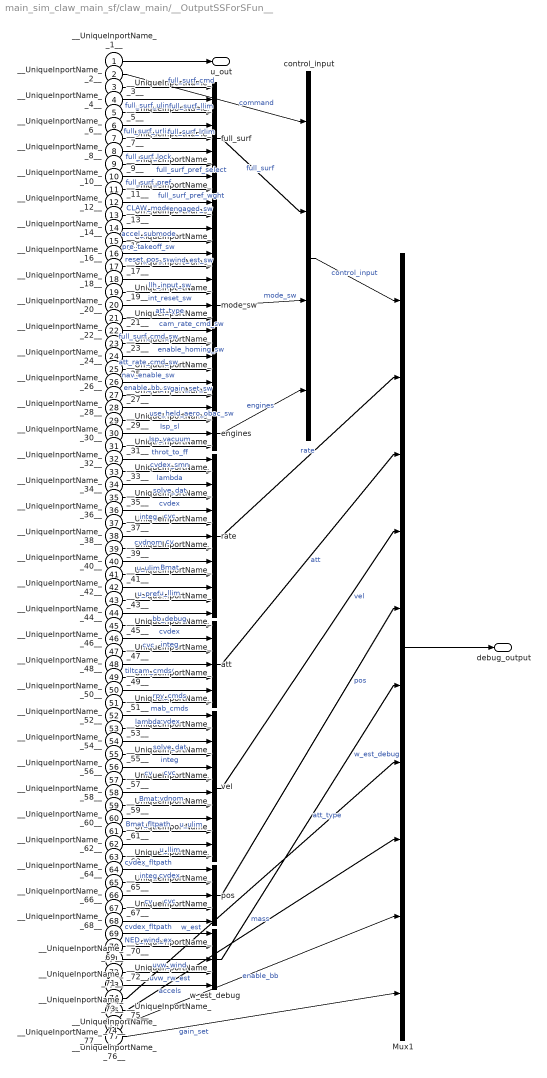
== system main_sim_claw_main_sf/claw_main/__OutputSSForSFun__ ==
  __UniqueInportName__1__ : Inport
  __UniqueInportName__2__ : Inport  Port=2
  __UniqueInportName__3__ : Inport  Port=3
  __UniqueInportName__4__ : Inport  Port=4
  __UniqueInportName__5__ : Inport  Port=5
  __UniqueInportName__6__ : Inport  Port=6
  __UniqueInportName__7__ : Inport  Port=7
  __UniqueInportName__8__ : Inport  Port=8
  __UniqueInportName__9__ : Inport  Port=9
  __UniqueInportName__10__ : Inport  Port=10
  __UniqueInportName__11__ : Inport  Port=11
  __UniqueInportName__12__ : Inport  Port=12
  __UniqueInportName__13__ : Inport  Port=13
  __UniqueInportName__14__ : Inport  Port=14
  __UniqueInportName__15__ : Inport  Port=15
  __UniqueInportName__16__ : Inport  Port=16
  __UniqueInportName__17__ : Inport  Port=17
  __UniqueInportName__18__ : Inport  Port=18
  __UniqueInportName__19__ : Inport  Port=19
  __UniqueInportName__20__ : Inport  Port=20
  __UniqueInportName__21__ : Inport  Port=21
  __UniqueInportName__22__ : Inport  Port=22
  __UniqueInportName__23__ : Inport  Port=23
  __UniqueInportName__24__ : Inport  Port=24
  __UniqueInportName__25__ : Inport  Port=25
  __UniqueInportName__26__ : Inport  Port=26
  __UniqueInportName__27__ : Inport  Port=27
  __UniqueInportName__28__ : Inport  Port=28
  __UniqueInportName__29__ : Inport  Port=29
  __UniqueInportName__30__ : Inport  Port=30
  __UniqueInportName__31__ : Inport  Port=31
  __UniqueInportName__32__ : Inport  Port=32
  __UniqueInportName__33__ : Inport  Port=33
  __UniqueInportName__34__ : Inport  Port=34
  __UniqueInportName__35__ : Inport  Port=35
  __UniqueInportName__36__ : Inport  Port=36
  __UniqueInportName__37__ : Inport  Port=37
  __UniqueInportName__38__ : Inport  Port=38
  __UniqueInportName__39__ : Inport  Port=39
  __UniqueInportName__40__ : Inport  Port=40
  __UniqueInportName__41__ : Inport  Port=41
  __UniqueInportName__42__ : Inport  Port=42
  __UniqueInportName__43__ : Inport  Port=43
  __UniqueInportName__44__ : Inport  Port=44
  __UniqueInportName__45__ : Inport  Port=45
  __UniqueInportName__46__ : Inport  Port=46
  __UniqueInportName__47__ : Inport  Port=47
  __UniqueInportName__48__ : Inport  Port=48
  __UniqueInportName__49__ : Inport  Port=49
  __UniqueInportName__50__ : Inport  Port=50
  __UniqueInportName__51__ : Inport  Port=51
  __UniqueInportName__52__ : Inport  Port=52
  __UniqueInportName__53__ : Inport  Port=53
  __UniqueInportName__54__ : Inport  Port=54
  __UniqueInportName__55__ : Inport  Port=55
  __UniqueInportName__56__ : Inport  Port=56
  __UniqueInportName__57__ : Inport  Port=57
  __UniqueInportName__58__ : Inport  Port=58
  __UniqueInportName__59__ : Inport  Port=59
  __UniqueInportName__60__ : Inport  Port=60
  __UniqueInportName__61__ : Inport  Port=61
  __UniqueInportName__62__ : Inport  Port=62
  __UniqueInportName__63__ : Inport  Port=63
  __UniqueInportName__64__ : Inport  Port=64
  __UniqueInportName__65__ : Inport  Port=65
  __UniqueInportName__66__ : Inport  Port=66
  __UniqueInportName__67__ : Inport  Port=67
  __UniqueInportName__68__ : Inport  Port=68
  __UniqueInportName__69__ : Inport  Port=69
  __UniqueInportName__70__ : Inport  Port=70
  __UniqueInportName__71__ : Inport  Port=71
  __UniqueInportName__72__ : Inport  Port=72
  __UniqueInportName__73__ : Inport  Port=73
  __UniqueInportName__74__ : Inport  Port=74
  __UniqueInportName__75__ : Inport  Port=75
  __UniqueInportName__76__ : Inport  Port=76
  __UniqueInportName__77__ : Inport  Port=77
  Mux1 : BusCreator  Inputs=10
  att : BusCreator  Inputs=7
  control_input : BusCreator
  engines : BusCreator  Inputs=3
  full_surf : BusCreator  Inputs=9
  mode_sw : BusCreator  Inputs=17
  pos : BusCreator  Inputs=5
  rate : BusCreator  Inputs=13
  vel : BusCreator  Inputs=12
  w_est_debug : BusCreator  Inputs=5
  u_out : Outport  OutDataType=sfix(16)  OutScaling=2^0
  debug_output : Outport  Port=2  OutDataType=sfix(16)  OutScaling=2^0
  wires:
  __UniqueInportName__1__/1 -> u_out/1
  __UniqueInportName__3__/1 -> full_surf/1  "full_surf_cmd"
  __UniqueInportName__4__/1 -> full_surf/2  "full_surf_ulim"
  __UniqueInportName__5__/1 -> full_surf/3  "full_surf_llim"
  __UniqueInportName__6__/1 -> full_surf/4  "full_surf_urlim"
  __UniqueInportName__7__/1 -> full_surf/5  "full_surf_lrlim"
  __UniqueInportName__8__/1 -> full_surf/6  "full_surf_lock"
  __UniqueInportName__9__/1 -> full_surf/7  "full_surf_pref_select"
  __UniqueInportName__10__/1 -> full_surf/8  "full_surf_pref"
  __UniqueInportName__11__/1 -> full_surf/9  "full_surf_pref_wght"
  __UniqueInportName__12__/1 -> mode_sw/1  "CLAW_mode"
  __UniqueInportName__13__/1 -> mode_sw/2  "engaged_sw"
  __UniqueInportName__14__/1 -> mode_sw/3  "accel_submode"
  __UniqueInportName__15__/1 -> mode_sw/4  "pre_takeoff_sw"
  __UniqueInportName__16__/1 -> mode_sw/5  "reset_pos_sw"
  __UniqueInportName__17__/1 -> mode_sw/6  "wind_est_sw"
  __UniqueInportName__18__/1 -> mode_sw/7  "llh_input_sw"
  __UniqueInportName__19__/1 -> mode_sw/8  "int_reset_sw"
  __UniqueInportName__20__/1 -> mode_sw/9  "att_type"
  __UniqueInportName__21__/1 -> mode_sw/10  "cam_rate_cmd_sw"
  __UniqueInportName__22__/1 -> mode_sw/11  "full_surf_cmd_sw"
  __UniqueInportName__23__/1 -> mode_sw/12  "enable_homing_sw"
  __UniqueInportName__24__/1 -> mode_sw/13  "att_rate_cmd_sw"
  __UniqueInportName__25__/1 -> mode_sw/14  "nav_enable_sw"
  __UniqueInportName__26__/1 -> mode_sw/15  "enable_bb_sw"
  __UniqueInportName__27__/1 -> mode_sw/16  "gain_set_sw"
  __UniqueInportName__28__/1 -> mode_sw/17  "use_held_aero_obac_sw"
  __UniqueInportName__29__/1 -> engines/1  "Isp_sl"
  __UniqueInportName__30__/1 -> engines/2  "Isp_vacuum"
  __UniqueInportName__31__/1 -> engines/3  "throt_to_ff"
  __UniqueInportName__2__/1 -> control_input/1  "command"
  full_surf/1 -> control_input/2  "full_surf"
  mode_sw/1 -> control_input/3  "mode_sw"
  engines/1 -> control_input/4  "engines"
  __UniqueInportName__32__/1 -> rate/1  "cvdex_smn"
  __UniqueInportName__33__/1 -> rate/2  "lambda"
  __UniqueInportName__34__/1 -> rate/3  "solve_dat"
  __UniqueInportName__35__/1 -> rate/4  "cvdex"
  __UniqueInportName__36__/1 -> rate/5  "cvc"
  __UniqueInportName__37__/1 -> rate/6  "integ"
  __UniqueInportName__38__/1 -> rate/7  "cv"
  __UniqueInportName__39__/1 -> rate/8  "cvdnom"
  __UniqueInportName__40__/1 -> rate/9  "Bmat"
  __UniqueInportName__41__/1 -> rate/10  "u_ulim"
  __UniqueInportName__42__/1 -> rate/11  "u_llim"
  __UniqueInportName__43__/1 -> rate/12  "u_pref"
  __UniqueInportName__44__/1 -> rate/13  "bb_debug"
  __UniqueInportName__45__/1 -> att/1  "cvdex"
  __UniqueInportName__46__/1 -> att/2  "integ"
  __UniqueInportName__47__/1 -> att/3  "cvc"
  __UniqueInportName__48__/1 -> att/4  "cv"
  __UniqueInportName__49__/1 -> att/5  "tiltcam_cmds"
  __UniqueInportName__50__/1 -> att/6  "rpy_cmds"
  __UniqueInportName__51__/1 -> att/7  "mab_cmds"
  __UniqueInportName__52__/1 -> vel/1  "cvdex"
  __UniqueInportName__53__/1 -> vel/2  "lambda"
  __UniqueInportName__54__/1 -> vel/3  "solve_dat"
  __UniqueInportName__55__/1 -> vel/4  "integ"
  __UniqueInportName__56__/1 -> vel/5  "cvc"
  __UniqueInportName__57__/1 -> vel/6  "cv"
  __UniqueInportName__58__/1 -> vel/7  "cvdnom"
  __UniqueInportName__59__/1 -> vel/8  "Bmat"
  __UniqueInportName__60__/1 -> vel/9  "Bmat_fltpath"
  __UniqueInportName__61__/1 -> vel/10  "u_ulim"
  __UniqueInportName__62__/1 -> vel/11  "u_llim"
  __UniqueInportName__63__/1 -> vel/12  "cvdex_fltpath"
  __UniqueInportName__64__/1 -> pos/1  "cvdex"
  __UniqueInportName__65__/1 -> pos/2  "integ"
  __UniqueInportName__66__/1 -> pos/3  "cvc"
  __UniqueInportName__67__/1 -> pos/4  "cv"
  __UniqueInportName__68__/1 -> pos/5  "cvdex_fltpath"
  __UniqueInportName__69__/1 -> w_est_debug/1  "w_est"
  __UniqueInportName__70__/1 -> w_est_debug/2  "NED_wind_ex"
  __UniqueInportName__71__/1 -> w_est_debug/3  "uvw_wind"
  __UniqueInportName__72__/1 -> w_est_debug/4  "uvw_rw_est"
  __UniqueInportName__73__/1 -> w_est_debug/5  "accels"
  control_input/1 -> Mux1/1  "control_input"
  rate/1 -> Mux1/2  "rate"
  att/1 -> Mux1/3  "att"
  vel/1 -> Mux1/4  "vel"
  pos/1 -> Mux1/5  "pos"
  w_est_debug/1 -> Mux1/6  "w_est_debug"
  __UniqueInportName__74__/1 -> Mux1/7  "att_type"
  __UniqueInportName__75__/1 -> Mux1/8  "mass"
  __UniqueInportName__76__/1 -> Mux1/9  "enable_bb"
  __UniqueInportName__77__/1 -> Mux1/10  "gain_set"
  Mux1/1 -> debug_output/1

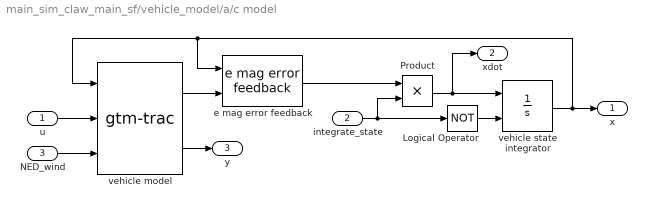
== system main_sim_claw_main_sf/vehicle_model/a/c model ==
  u : Inport  OutDataType=sfix(16)  OutScaling=2^0
  integrate_state : Inport  Port=2  OutDataType=sfix(16)  OutScaling=2^0
  NED_wind : Inport  Port=3  OutDataType=sfix(16)  OutScaling=2^0
  Logical Operator : Logic  Operator=NOT  AllPortsSameDT=off  OutDataTypeMode=boolean  OutDataTypeStr=boolean
  Product : Product  OutDataType=sfix(16)  OutScaling=2^0  RndMeth=Zero
  e mag error feedback : model_lib/e mag error feedback  SystemSampleTime=-1
  vehicle model : models/gtm-trac  SystemSampleTime=-1  vehicle_params=trac_params
  vehicle state integrator : Integrator  ExternalReset=level  InitialCondition=x_trac_IC
  x : Outport  OutDataType=sfix(16)  OutScaling=2^0
  xdot : Outport  Port=2  OutDataType=sfix(16)  OutScaling=2^0
  y : Outport  Port=3  OutDataType=sfix(16)  OutScaling=2^0
  wires:
  u/1 -> vehicle model/2
  vehicle state integrator/1 -> x/1, vehicle model/1, e mag error feedback/1
  integrate_state/1 -> Logical Operator/1, Product/2
  Product/1 -> xdot/1, vehicle state integrator/1
  Logical Operator/1 -> vehicle state integrator/2
  NED_wind/1 -> vehicle model/3
  vehicle model/2 -> y/1
  e mag error feedback/1 -> Product/1
  vehicle model/1 -> e mag error feedback/2

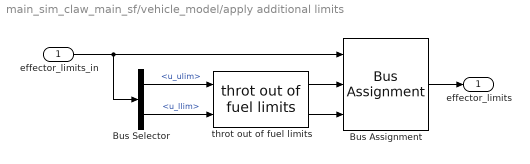
== system main_sim_claw_main_sf/vehicle_model/apply additional limits ==
  effector_limits_in : Inport  OutDataType=sfix(16)  OutScaling=2^0
  Bus Assignment : BusAssignment  AssignedSignals=u_ulim,u_llim
  Bus Selector : BusSelector  OutputSignals=u_ulim,u_llim
  throt out of fuel limits : model_lib/throt out of fuel limits  SystemSampleTime=-1
  effector_limits : Outport  OutDataType=sfix(16)  OutScaling=2^0
  wires:
  effector_limits_in/1 -> Bus Assignment/1, Bus Selector/1
  Bus Selector/1 -> throt out of fuel limits/1  "<u_ulim>"
  Bus Selector/2 -> throt out of fuel limits/2  "<u_llim>"
  Bus Assignment/1 -> effector_limits/1
  throt out of fuel limits/1 -> Bus Assignment/2
  throt out of fuel limits/2 -> Bus Assignment/3

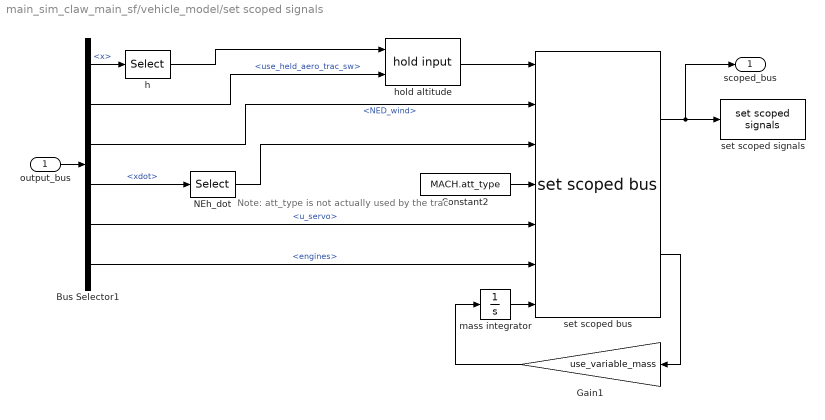
== system main_sim_claw_main_sf/vehicle_model/set scoped signals ==
  note: Note: att_type is not actually
      | used by the trac
  output_bus : Inport  OutDataType=sfix(16)  OutScaling=2^0
  Bus Selector1 : BusSelector  OutputSignals=x,use_held_aero_trac_sw,NED_wind,xdot,u_servo,engines
  Constant2 : Constant  Value=MACH.att_type  OutDataType=sfix(16)  OutScaling=2^0
  Gain1 : Gain  Orientation=left  Gain=use_variable_mass  ParameterDataType=sfix(16)  ParameterScaling=2^0  OutDataType=sfix(16)  OutScaling=2^0
  NEh_dot : Selector  InputPortWidth=trac_params.num_x  IndexOptions=Index vector (dialog)  Indices=MACH.NEh_idx  OutputSizes=1
  h : Selector  InputPortWidth=MACH.num_x  IndexOptions=Index vector (dialog)  Indices=MACH.NEh_idx(3)  OutputSizes=1
  hold altitude : model_lib/hold input  SystemSampleTime=-1
  mass integrator : Integrator  InitialCondition=trac_params.mass_IC
  set scoped bus : model_lib/set scoped bus  SystemSampleTime=-1  vehicle_params=trac_params
  set scoped signals : model_lib/set scoped signals  SystemSampleTime=-1
  scoped_bus : Outport  OutDataType=sfix(16)  OutScaling=2^0
  wires:
  Bus Selector1/1 -> h/1  "<x>"
  NEh_dot/1 -> set scoped bus/3
  Bus Selector1/3 -> set scoped bus/2  "<NED_wind>"
  Bus Selector1/5 -> set scoped bus/5  "<u_servo>"
  mass integrator/1 -> set scoped bus/7
  set scoped bus/2 -> Gain1/1
  Gain1/1 -> mass integrator/1
  hold altitude/1 -> set scoped bus/1
  h/1 -> hold altitude/1
  Bus Selector1/2 -> hold altitude/2  "<use_held_aero_trac_sw>"
  set scoped bus/1 -> set scoped signals/1, scoped_bus/1
  Constant2/1 -> set scoped bus/4
  Bus Selector1/4 -> NEh_dot/1  "<xdot>"
  output_bus/1 -> Bus Selector1/1
  Bus Selector1/6 -> set scoped bus/6  "<engines>"

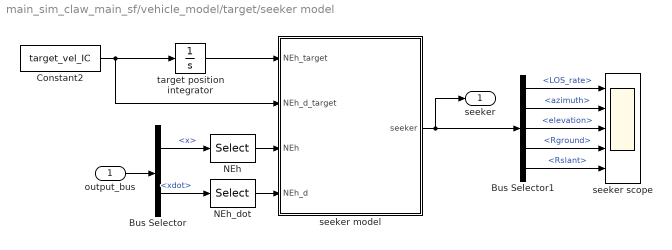
== system main_sim_claw_main_sf/vehicle_model/target/seeker model ==
  output_bus : Inport  OutDataType=sfix(16)  OutScaling=2^0
  Bus Selector : BusSelector  OutputSignals=x,xdot
  Bus Selector1 : BusSelector  OutputSignals=LOS_rate,aux_info.azimuth,aux_info.elevation,aux_info.Rground,aux_info.Rslant
  Constant2 : Constant  Value=target_vel_IC  OutDataType=sfix(16)  OutScaling=2^0
  NEh : Selector  InputPortWidth=MACH.num_x  IndexOptions=Index vector (dialog)  Indices=MACH.NEh_idx  OutputSizes=1
  NEh_dot : Selector  InputPortWidth=MACH.num_x  IndexOptions=Index vector (dialog)  Indices=MACH.NEh_idx  OutputSizes=1
  seeker model : Subsystem
  seeker scope : Scope  NumInputPorts=5
      settings: YMin=-1.75~-3.5~-1.75~0~0  YMax=0.25~0.5~0~450000~550000
  target position integrator : Integrator  InitialCondition=target_pos_IC
  seeker : Outport  OutDataType=sfix(16)  OutScaling=2^0
  wires:
  Constant2/1 -> target position integrator/1, seeker model/2(NEh_d_target)
  target position integrator/1 -> seeker model/1(NEh_target)
  NEh/1 -> seeker model/3(NEh)
  NEh_dot/1 -> seeker model/4(NEh_d)
  seeker model/1(seeker) -> seeker/1, Bus Selector1/1
  output_bus/1 -> Bus Selector/1
  Bus Selector/1 -> NEh/1  "<x>"
  Bus Selector/2 -> NEh_dot/1  "<xdot>"
  Bus Selector1/2 -> seeker scope/2  "<azimuth>"
  Bus Selector1/3 -> seeker scope/3  "<elevation>"
  Bus Selector1/4 -> seeker scope/4  "<Rground>"
  Bus Selector1/5 -> seeker scope/5  "<Rslant>"
  Bus Selector1/1 -> seeker scope/1  "<LOS_rate>"
